simulink model "Arduino_Spider_Demo"  (R2016a)
settings: Solver=FixedStepAuto  StartTime=0.0  StopTime=inf  RelTol=1e-3
libraries: arduinolib x13
settings Model: SimulationMode=external  ExtModeTrigDuration=2  Creator=Eric MARCHAND  LastModifiedBy=nickchoi
settings OptimizationCC: OptimizeModelRefInitCode=on  LifeSpan=Inf  MaxStackSize=64
settings HardwareCC: ProdBitPerInt=16  ProdBitPerPointer=16  ProdLargestAtomicFloat=None  ProdWordSize=8  ProdHWDeviceType=Atmel->AVR
settings RTWCC: SystemTargetFile=ert.tlc  HardwareBoard=Arduino Mega 2560  TemplateMakefile=ert_default_tmf  GenerateReport=on  Toolchain=Arduino AVR v1.6.1  BuildConfiguration=Faster Runs  IncludeHyperlinkInReport=on  LaunchReport=on  GenerateTraceInfo=on  GenerateTraceReport=on  GenerateTraceReportSl=on  GenerateTraceReportSf=on  GenerateTraceReportEml=on
settings CodeAppCC: ForceParamTrailComments=on  IgnoreCustomStorageClasses=off  OperatorAnnotations=on  SimulinkDataObjDesc=on  SFDataObjDesc=on  MATLABFcnDesc=on  InsertBlockDesc=on  MATLABSourceComments=on
settings ERTTargetCC: SupportContinuousTime=on  SupportNonInlinedSFcns=on  SupportVariableSizeSignals=on

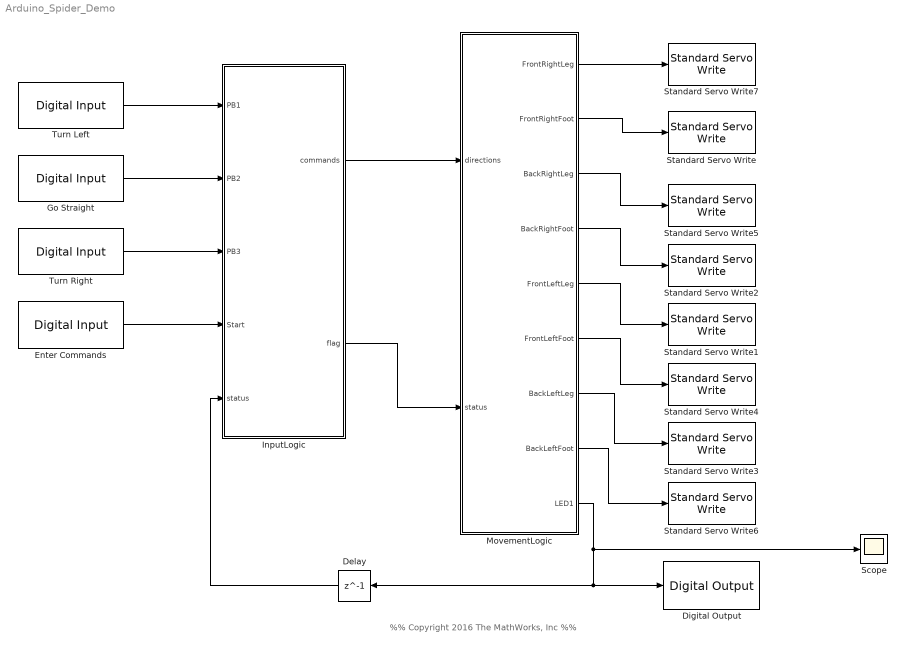
== system Arduino_Spider_Demo ==
  note: %% Copyright 2016 The MathWorks, Inc %%
  Delay : Delay  DelayLength=1  InitialCondition=0
  Digital Output : arduinolib/Digital Output  pinNumber=30  blockPlatform=arduino
  Enter Commands : arduinolib/Digital Input  pinNumber=22  sampleTime=.1  blockPlatform=arduino
  Go Straight : arduinolib/Digital Input  pinNumber=26  sampleTime=.1  blockPlatform=arduino
  InputLogic : Stateflow chart  TreatAsAtomicUnit=on
  "MovementLogic " : Stateflow chart  TreatAsAtomicUnit=on
  Scope : Scope
  Standard Servo Write : arduinolib/Standard Servo Write  pinNumber=3  blockPlatform=arduino
  Standard Servo Write1 : arduinolib/Standard Servo Write  pinNumber=6  blockPlatform=arduino
  Standard Servo Write2 : arduinolib/Standard Servo Write  pinNumber=5  blockPlatform=arduino
  Standard Servo Write3 : arduinolib/Standard Servo Write  pinNumber=9  blockPlatform=arduino
  Standard Servo Write4 : arduinolib/Standard Servo Write  pinNumber=7  blockPlatform=arduino
  Standard Servo Write5 : arduinolib/Standard Servo Write  pinNumber=4  blockPlatform=arduino
  Standard Servo Write6 : arduinolib/Standard Servo Write  pinNumber=8  blockPlatform=arduino
  Standard Servo Write7 : arduinolib/Standard Servo Write  pinNumber=2  blockPlatform=arduino
  Turn Left : arduinolib/Digital Input  pinNumber=28  sampleTime=.1  blockPlatform=arduino
  Turn Right : arduinolib/Digital Input  pinNumber=24  sampleTime=.1  blockPlatform=arduino
  wires:
  "MovementLogic "/8(BackLeftFoot) -> Standard Servo Write6/1
  "MovementLogic "/7(BackLeftLeg) -> Standard Servo Write3/1
  "MovementLogic "/6(FrontLeftFoot) -> Standard Servo Write4/1
  "MovementLogic "/5(FrontLeftLeg) -> Standard Servo Write1/1
  "MovementLogic "/4(BackRightFoot) -> Standard Servo Write2/1
  "MovementLogic "/1(FrontRightLeg) -> Standard Servo Write7/1
  "MovementLogic "/2(FrontRightFoot) -> Standard Servo Write/1
  "MovementLogic "/3(BackRightLeg) -> Standard Servo Write5/1
  Turn Left/1 -> InputLogic/1(PB1)
  Go Straight/1 -> InputLogic/2(PB2)
  Turn Right/1 -> InputLogic/3(PB3)
  Enter Commands/1 -> InputLogic/4(Start)
  "MovementLogic "/9(LED1) -> Delay/1, Digital Output/1, Scope/1
  Delay/1 -> InputLogic/5(status)
  InputLogic/2(flag) -> "MovementLogic "/2(status)
  InputLogic/1(commands) -> "MovementLogic "/1(directions)

== stateflow chart Arduino_Spider_Demo/InputLogic ==
  state INIT
    entry:
    progress = uint8(1);
    route = [0 0 0 0 0 0 0 0 0 0];
    commands = [0 0 0 0 0 0 0 0 0 0];
    full = false;
    flag = false;
  state WaitForInputs
  state PB1
    entry:
    route(progress) = 1;
    progress = progress + 1;
  state WaitToRefresh
  state PB3
    entry:
    route(progress) = 3;
    progress = progress + 1;
  state PB2
    entry:
    route(progress) = 2;
    progress = progress + 1;
  state Evaluate
    entry:
    if (progress == 11) || Start
    commands = route;
    flag = true;
    full = true;
    end
  (default) -> INIT
  WaitToRefresh -> INIT : [after(3.5, sec) && ~status]
  INIT -> WaitForInputs : [~status]
  WaitForInputs -> PB1 [order 2] : [xor([PB1], [PB2]) && xor([PB1],[PB3]) ]
  WaitForInputs -> PB3 [order 1] : [xor([PB3], [PB2]) && xor([PB3],[PB1]) ]
  WaitForInputs -> Evaluate [order 4] : [Start]
  Evaluate -> WaitForInputs [order 2] : [~(PB1 || PB2 || PB3) && ~(Start || full == true)]
  WaitForInputs -> PB2 [order 3] : [xor([PB2], [PB3]) && xor([PB2],[PB1]) ]
  Evaluate -> WaitToRefresh [order 1] : [full ]
  PB1 -> Evaluate
  PB2 -> Evaluate
  PB3 -> Evaluate
  data: commands output size=[1 10]; PB1 input; PB2 input; PB3 input; Start input; route local size=[1 10]; progress local uint8; full local boolean; status input; flag output

== stateflow chart Arduino_Spider_Demo/MovementLogic  ==
  state INIT
    entry:
    LED1 = 0;
    FrontRightLeg=90; FrontRightFoot=10;
    FrontLeftLeg=90; FrontLeftFoot=10;
    BackRightLeg=100; BackRightFoot=10;
    BackLeftLeg=80; BackLeftFoot=10;
  state WaitingForInput
    entry:
    LED1 = 0;
  state Init2
    entry:
    LED1 = 1;
    progress = uint8(1); path = directions;
  state TurnLeft
    entry:
    FrontRightLeg=90;
    FrontRightFoot=10;
    BackRightLeg=140;
    BackRightFoot=10;
    BackLeftLeg = 150;
    FrontLeftLeg=170;
  state PickDirection
    exit:
    progress = progress + 1;
  state TurnRight
    entry:
    FrontRightLeg=10;
    FrontRightFoot=20;
    BackRightLeg=10;
    BackRightFoot=10;
    BackLeftLeg =50;
    FrontLeftLeg=70;
  state Reset2
    entry:
    FrontRightLeg=90; FrontRightFoot=10;
    FrontLeftLeg=90; FrontLeftFoot=10;
    BackRightLeg=100; BackRightFoot=10;
    BackLeftLeg=80; BackLeftFoot=10;
  state TurnLeft1
    entry:
    FrontRightLeg=90;
    BackRightLeg=90;
    BackLeftLeg=90;
  state TurnRight1
    entry:
    FrontLeftLeg=90;
    BackRightLeg=90;
    BackLeftLeg=90;
  state Forward2
    state Start4
      entry:
      FrontRightLeg=40;
      FrontRightFoot = 40;
      BackLeftLeg=130;
    state Start5
      entry:
      BackLeftLeg=90;
      FrontRightLeg=90;
      FrontRightFoot = 10;
    (default) -> Start4
    Start4 -> Start5 : after(.25,sec)
  state Forward
    state Start
      entry:
      FrontLeftLeg=140;
      FrontLeftFoot = 40;
      BackRightLeg = 50;
    state Start2
      entry:
      FrontLeftLeg=90;
      FrontLeftFoot = 10;
      BackRightLeg = 90;
    (default) -> Start
    Start -> Start2 : after(0.25,sec)
  (default) -> INIT
  WaitingForInput -> INIT : after(1,sec)
  INIT -> Init2 : [status]
  PickDirection -> WaitingForInput [order 2] : [progress == 11]
  Init2 -> PickDirection : [after(2,sec)]
  PickDirection -> PickDirection [order 5] : [path(progress) == 0]
  PickDirection -> TurnLeft [order 4] : [after(.25,sec) && path(progress) == 1]
  PickDirection -> TurnRight [order 3] : [after(.25,sec) && path(progress) == 3]
  PickDirection -> Forward [order 1] : [after(.25,sec) && path(progress) == 2]
  Reset2 -> PickDirection : after(0.75,sec)
  TurnLeft -> TurnLeft1 : after(1,sec)
  TurnRight -> TurnRight1 : after(1,sec)
  TurnLeft1 -> Reset2 : after(.5,sec)
  TurnRight1 -> Reset2 : after(.5,sec)
  Forward2 -> Reset2 : after(0.5,sec)
  Forward -> Forward2 : after(.5,sec)
  data: FrontRightLeg output; FrontRightFoot output; BackRightLeg output; BackRightFoot output; FrontLeftLeg output; FrontLeftFoot output; BackLeftLeg output; BackLeftFoot output; directions input; progress local uint8; path local size=[1 10]; LED1 output; status input
